simulink model "force_control"  (R2021a)
settings: Solver=FixedStepDiscrete  StartTime=0.0  StopTime=inf  FixedStep=0.001  RelTol=1e-3  EnableMultiTasking=on
PreLoadFcn:
  | demos_common_configs();
undefined symbols (not defined in the file): ddQ2_desired, ddQ4_desired, DiscIntNeverNeededParam, dQ2_desired, dQ4_desired, Q2_desired, Q4_desired, T
libraries: simulink x6, franka_simulink_library_misc x5, franka_simulink_library x4
settings Model: SimulationMode=external  ExtModeTrigDuration=10000  Creator=vasi_ko  LastModifiedBy=robohub
settings SolverCC: AlgebraicLoopSolver=TrustRegion
settings DataIOCC: LimitDataPoints=on  SaveFormat=Array  ReturnWorkspaceOutputs=off
settings OptimizationCC: DefaultParameterBehavior=Inlined  EnhancedBackFolding=on  PassReuseOutputArgsAs=Individual arguments  ZeroExternalMemoryAtStartup=off  ZeroInternalMemoryAtStartup=off  OptimizeBlockOrder=speed  DifferentSizesBufferReuse=on  OptimizationCustomize=off  EfficientTunableParamExpr=on
settings DebuggingCC: SolverPrmCheckMsg=warning  ParameterTunabilityLossMsg=error  SFUnexpectedBacktrackingDiag=warning  SFNoUnconditionalDefaultTransitionDiag=warning  SFExecutionAtInitializationDiag=none  SFMachineParentedDataDiag=warning  ArithmeticOperatorsInVariantConditions=warning
settings HardwareCC: ProdBitPerLong=64  ProdHWDeviceType=Intel->x86-64 (Linux 64)
settings ModelReferenceCC: PropagateSignalLabelsOutOfModel=off
settings SFSimCC: SimUseLocalCustomCode=off  MATLABDynamicMemAlloc=off  CustomCodeUndefinedFunction=UseInterfaceOnly  SimTargetLang=C++
settings RTWCC: SystemTargetFile=franka_emika_panda.tlc  GenCodeOnly=on  TemplateMakefile=ert_default_tmf  RTWVerbose=off  RTWUseLocalCustomCode=off  Toolchain=Franka Simulink | gmake (64-bit linux)  BuildConfiguration=Faster Runs  IncludeHyperlinkInReport=on  TargetLang=C++
settings CodeAppCC: ForceParamTrailComments=on  IgnoreCustomStorageClasses=off  OperatorAnnotations=on  SimulinkDataObjDesc=on  SFDataObjDesc=on  InsertBlockDesc=on
settings STFCustomTargetCC: TargetLangStandard=C99 (ISO)  MultiwordLength=256  GenerateSampleERTMain=on  ModelReferenceCompliant=off  CombineOutputUpdateFcns=on  ERTCustomFileBanners=on  SupportNonInlinedSFcns=off  RemoveResetFunc=on  MATLABClassNameForMDSCustomization=Simulink.SoftwareTarget.ERTCustomization  CPPClassGenCompliant=on  GRTInterface=off  SystemTargetFile=franka_emika_panda.tlc
settings ERTTargetCC: TargetLangStandard=C99 (ISO)  GenerateSampleERTMain=on  ModelReferenceCompliant=off  ParMdlRefBuildCompliant=off  CompOptLevelCompliant=off  ConcurrentExecutionCompliant=off  SupportContinuousTime=on  ModelStepFunctionPrototypeControlCompliant=off  ExtMode=on  ExtModeMexArgs='129.97.71.27' 0 17725  InlinedParameterPlacement=NonHierarchical  ERTCustomFileTemplate=franka_emika_panda_file_process.tlc
settings ConfigComp: CovMetricSettings=dw  CovSaveCumulativeToWorkspaceVar=on  CovSaveSingleToWorkspaceVar=on  CovExternalEMLEnable=off  CovSFcnEnable=off

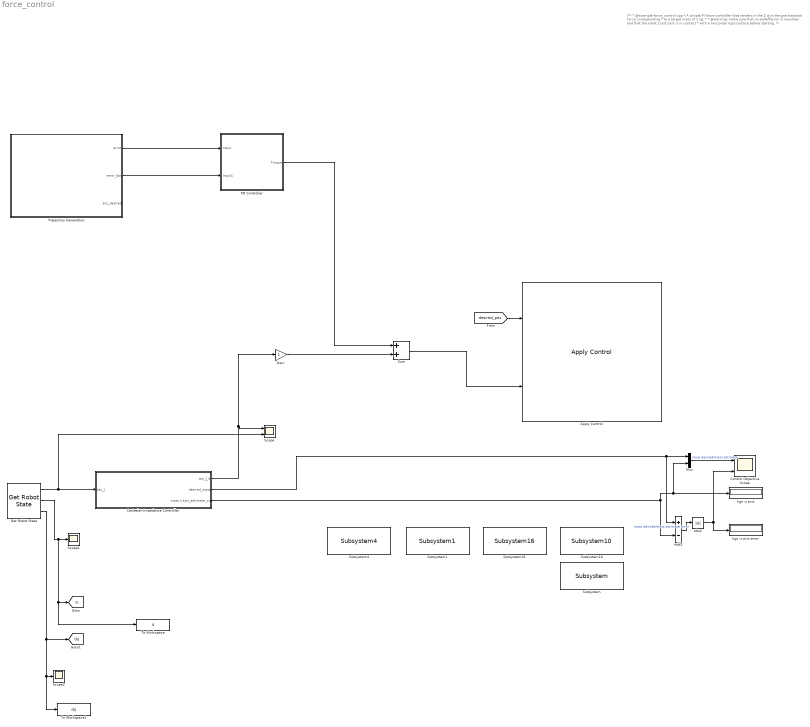
== system force_control ==
  note: /**
      |  * @example force_control.cpp
      |  * A simple PI force controller that renders in the Z axis the gravitational force corresponding
      |  * to a target mass of 1 kg.
      |  *
      |  * @warning: make sure that no endeffector is mounted and that the robot's last joint is in contact
      |  * with a horizontal rigid surface before starting.
      |  */
  Abs2 : Abs
  Add1 : Sum  Inputs=+-
  Apply Control : franka_simulink_library/Apply Control  robot_ip=robot_ip  gripper_attached=off  control_mode=Torque Control - Joint Positions  controller_choice=Joint Impedance Controller  elbow_control=on  collision_thresholds=100*ones(1,52)  joint_impedance=joint_impedance  cartesian_impedance=cartesian_impedance  load_inertia=load_inertia  EE_T_K=EE_T_K  init_joint_configuration_req=off  init_joint_configuration=[0.00392584915725334;-0.104076810189763;0.0404703493577216;-2.7334242600631;0.0113035300040543;2.63364770337236;0.372162046953987]
      settings: SourceProductName=Franka Emika
  Cartesian Impedance Controller : Subsystem
      mask Display:
      | disp('{\bf\fontsize{18}Force Controller}', 'texmode','on');
      | %
      | % block_icon('Controller')
      | %
      | port_label('input',1,'tau_J');
      | port_label('output',1,'tau_J_d');
      | port_label('output',2,'mass desired');
      | port_label('output',3,'mass estimate');
  Control Objective Scope : Scope  NumInputPorts=2
  Gain : Gain
  Get Robot State : franka_simulink_library/Get Robot State  robot_ip=robot_ip  signals_requested='tau_J q dq'
      settings: SourceProductName=Franka Emika
  Mux : Mux  Inputs=2
  PD Controller : Subsystem
  Scope : Scope  NumInputPorts=2
  Scope1 : Scope
  Scope2 : Scope
  Subsystem : franka_simulink_library_misc/Subsystem  SystemSampleTime=-1  VariantActivationTime=update diagram  Latency=0  AutoFrameSizeCalculation=off
  Subsystem1 : franka_simulink_library_misc/Subsystem1  SystemSampleTime=-1  VariantActivationTime=update diagram  Latency=0  AutoFrameSizeCalculation=off
  Subsystem10 : franka_simulink_library_misc/Subsystem10  SystemSampleTime=-1  VariantActivationTime=update diagram  Latency=0  AutoFrameSizeCalculation=off
  Subsystem16 : franka_simulink_library_misc/Subsystem16  SystemSampleTime=-1  VariantActivationTime=update diagram  Latency=0  AutoFrameSizeCalculation=off
  Subsystem4 : franka_simulink_library_misc/Subsystem4  SystemSampleTime=-1  VariantActivationTime=update diagram  Latency=0  AutoFrameSizeCalculation=off
  Sum : Sum
  To Workspace : ToWorkspace  VariableName=q  SaveFormat=Structure With Time  SampleTime=-1
  To Workspace1 : ToWorkspace  VariableName=dq  SaveFormat=Structure With Time  SampleTime=-1
  Trajectory Generation : Subsystem
  kgs -z axis : Display
  kgs -z axis error : Display
  tag scope: dq=global, q=global
  wires:
  Get Robot State/1 -> Scope/2, Cartesian Impedance Controller/1(tau_J)
  Mux/1 -> Control Objective Scope/1  "mass desired/mass estimate"
  Cartesian Impedance Controller/1(tau_J_d) -> Gain/1, Scope/1
  Cartesian Impedance Controller/2(desired_mass) -> Add1/1, Mux/1
  Cartesian Impedance Controller/3(mass z axis_estimate_out) -> kgs -z axis/1, Mux/2, Add1/2
  Add1/1 -> Abs2/1  "mass desired/mass estimate error"
  Abs2/1 -> kgs -z axis error/1, Control Objective Scope/2
  Get Robot State/3 -> [dq], To Workspace1/1, Scope2/1
  Trajectory Generation/2(error_dot) -> PD Controller/2(Input1)
  Trajectory Generation/1(error) -> PD Controller/1(Input)
  Get Robot State/2 -> [q], To Workspace/1, Scope1/1
  PD Controller/1(Torque) -> Sum/1
  Gain/1 -> Sum/2
  Sum/1 -> Apply Control/2
  [desired_pos] -> Apply Control/1

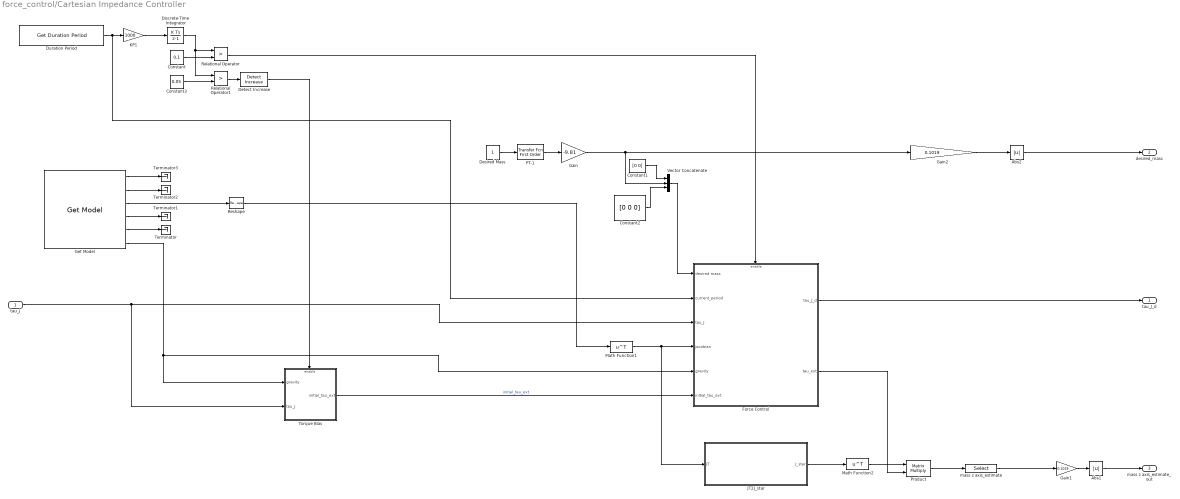
== system force_control/Cartesian Impedance Controller ==
  tau_J : Inport
  Abs1 : Abs
  Abs2 : Abs
  Constant : Constant  Value=0.1
  Constant1 : Constant  Value=[0 0]
  Constant2 : Constant  Value=[0 0 0]
  Constant3 : Constant  Value=0.05
  Desired Mass : Constant
  Detect Increase : simulink/Logic and Bit Operations/Detect Increase  vinit=0.0  OutDataTypeStr=boolean
  Discrete-Time Integrator : DiscreteIntegrator  SampleTime=-1  ICPrevOutput=DiscIntNeverNeededParam  ICPrevScaledInput=DiscIntNeverNeededParam
  Duration Period : franka_simulink_library/Get Duration Period  robot_ip=robot_ip
      settings: SourceProductName=Franka Emika
  Force Control : Subsystem
  Gain : Gain  Gain=-9.81
  Gain1 : Gain  Gain=0.1019
  Gain2 : Gain  Gain=0.1019
  Get Model : franka_simulink_library/Get Model  robot_ip=robot_ip
      settings: SourceProductName=Franka Emika
  JT2J_star : MATLAB Function  TreatAsAtomicUnit=on
  KP1 : Gain  Gain=1000
  Math Function1 : Math  Operator=transpose  SignedPower=on  SaturateOnIntegerOverflow=on
  Math Function2 : Math  Operator=transpose  SignedPower=on  SaturateOnIntegerOverflow=on
  PT-1 : simulink/Discrete/Transfer Fcn First Order  PoleZ=0.9988  ICPrevOutput=0.0  DoSatur=off
  Product : Product  Multiplication=Matrix(*)
  Relational Operator : RelationalOperator  Operator=>  OutDataTypeStr=boolean  RndMeth=Nearest
  Relational Operator1 : RelationalOperator  Operator=>  OutDataTypeStr=boolean  RndMeth=Nearest
  Reshape : Reshape  OutputDimensionality=Customize  OutputDimensions=[6,7]
  Terminator{,1..3} (4 alike) : Terminator
  Torque Bias : Subsystem
  Vector Concatenate : Concatenate  NumInputs=3
  mass z axis_estimate : Selector  InputPortWidth=6  IndexOptions=Index vector (dialog)  Indices=3  OutputSizes=1
  tau_J_d : Outport  VectorParamsAs1DForOutWhenUnconnected=off
  desired_mass : Outport  Port=2  VectorParamsAs1DForOutWhenUnconnected=off
  mass z axis_estimate_out : Outport  Port=3  VectorParamsAs1DForOutWhenUnconnected=off
  wires:
  Get Model/5 -> Terminator/1
  Get Model/4 -> Terminator1/1
  Get Model/3 -> Reshape/1
  tau_J/1 -> Force Control/3(tau_J), Torque Bias/2(tau_J)
  Discrete-Time Integrator/1 -> Relational Operator1/1, Relational Operator/1
  Constant/1 -> Relational Operator/2
  KP1/1 -> Discrete-Time Integrator/1
  Constant1/1 -> Vector Concatenate/1
  Constant2/1 -> Vector Concatenate/3
  Desired Mass/1 -> PT-1/1
  Gain/1 -> Vector Concatenate/2, Gain2/1
  Force Control/1(tau_J_d) -> tau_J_d/1
  Torque Bias/1(initial_tau_ext) -> Force Control/6(initial_tau_ext)  "initial_tau_ext"
  Get Model/6 -> Torque Bias/1(gravity), Force Control/5(gravity)
  Relational Operator/1 -> Force Control/Enable
  Reshape/1 -> Math Function1/1
  Duration Period/1 -> KP1/1, Force Control/2(current_period)
  Constant3/1 -> Relational Operator1/2
  Relational Operator1/1 -> Detect Increase/1
  Detect Increase/1 -> Torque Bias/Enable
  Vector Concatenate/1 -> Force Control/1(desired mass)
  PT-1/1 -> Gain/1
  Force Control/2(tau_ext) -> Product/2
  Gain1/1 -> Abs1/1
  Gain2/1 -> Abs2/1
  Abs1/1 -> mass z axis_estimate_out/1
  Abs2/1 -> desired_mass/1
  Get Model/1 -> Terminator3/1
  mass z axis_estimate/1 -> Gain1/1
  Get Model/2 -> Terminator2/1
  Product/1 -> mass z axis_estimate/1
  Math Function1/1 -> JT2J_star/1(JT), Force Control/4(Jacobian)
  JT2J_star/1(J_star) -> Math Function2/1
  Math Function2/1 -> Product/1

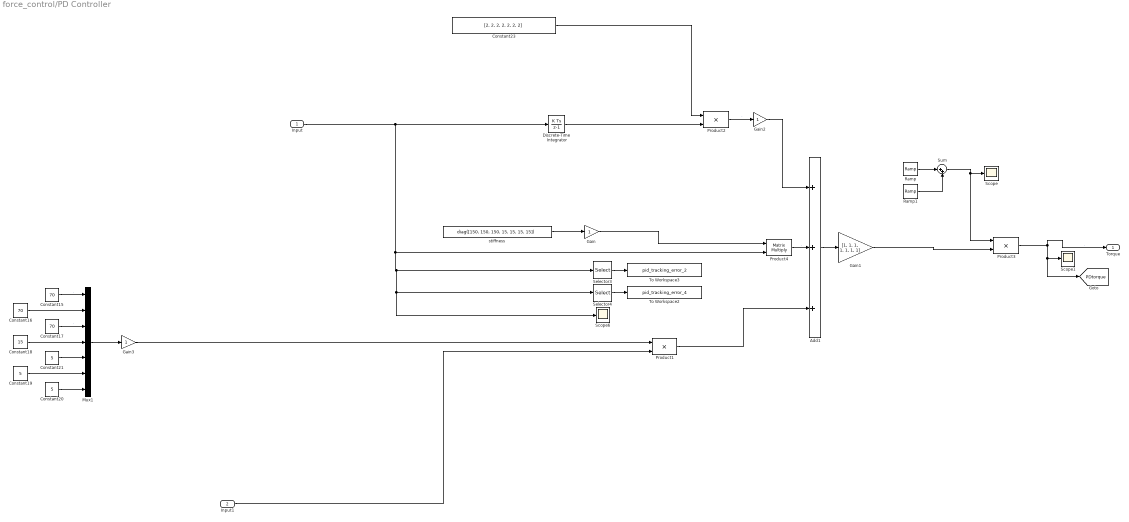
== system force_control/PD Controller ==
  Input : Inport
  Input1 : Inport  Port=2
  Add1 : Sum  Inputs=+++
  Constant15 : Constant  Value=70
  Constant16 : Constant  Value=70
  Constant17 : Constant  Value=70
  Constant18 : Constant  Value=15
  Constant19 : Constant  Value=5
  Constant20 : Constant  Value=5
  Constant21 : Constant  Value=5
  Constant23 : Constant  Value=[2, 2, 2, 2, 2, 2, 2]
  Discrete-Time Integrator : DiscreteIntegrator  SampleTime=-1  ICPrevOutput=DiscIntNeverNeededParam  ICPrevScaledInput=DiscIntNeverNeededParam
  Gain : Gain
  Gain1 : Gain  Gain=[1, 1, 1, 1, 1, 1, 1]
  Gain2 : Gain
  Gain3 : Gain
  Mux1 : Mux  Inputs=7
  Product1 : Product
  Product2 : Product
  Product3 : Product
  Product4 : Product  Multiplication=Matrix(*)
  Ramp : simulink/Sources/Ramp  slope=0.1  start=0  InitialOutput=0
  Ramp1 : simulink/Sources/Ramp  slope=-0.1  start=10  InitialOutput=0
  Scope : Scope
  Scope1 : Scope
  Scope6 : Scope
  Selector3 : Selector  InputPortWidth=7  IndexOptions=Index vector (dialog)  Indices=[2]  OutputSizes=1
  Selector4 : Selector  InputPortWidth=7  IndexOptions=Index vector (dialog)  Indices=[4]  OutputSizes=1
  Sum : Sum  Inputs=|++
  To Workspace2 : ToWorkspace  VariableName=pid_tracking_error_4  SaveFormat=Structure With Time  SampleTime=-1
  To Workspace3 : ToWorkspace  VariableName=pid_tracking_error_2  SaveFormat=Structure With Time  SampleTime=-1
  stiffness : Constant  Value=diag([150, 150, 150, 15, 15, 15, 15])  VectorParams1D=off
  Torque : Outport
  tag scope: PDtorque=global
  wires:
  Product4/1 -> Add1/2  "."
  Mux1/1 -> Gain3/1
  Constant16/1 -> Mux1/2
  Constant18/1 -> Mux1/4
  Constant19/1 -> Mux1/6
  Constant20/1 -> Mux1/7
  Constant21/1 -> Mux1/5
  Constant15/1 -> Mux1/1  "."
  Constant17/1 -> Mux1/3  "."
  Product1/1 -> Add1/3
  Add1/1 -> Gain1/1
  Constant23/1 -> Product2/1
  Product2/1 -> Gain2/1  "."
  Discrete-Time Integrator/1 -> Product2/2
  Selector4/1 -> To Workspace2/1
  Selector3/1 -> To Workspace3/1
  stiffness/1 -> Gain/1
  Gain2/1 -> Add1/1
  Gain3/1 -> Product1/1
  Input/1 -> Scope6/1, Selector4/1, Selector3/1, Product4/2, Discrete-Time Integrator/1
  Input1/1 -> Product1/2
  Gain/1 -> Product4/1
  Ramp/1 -> Sum/1
  Ramp1/1 -> Sum/2
  Gain1/1 -> Product3/2
  Product3/1 -> Torque/1, Scope1/1, [PDtorque]  "."
  Sum/1 -> Scope/1, Product3/1

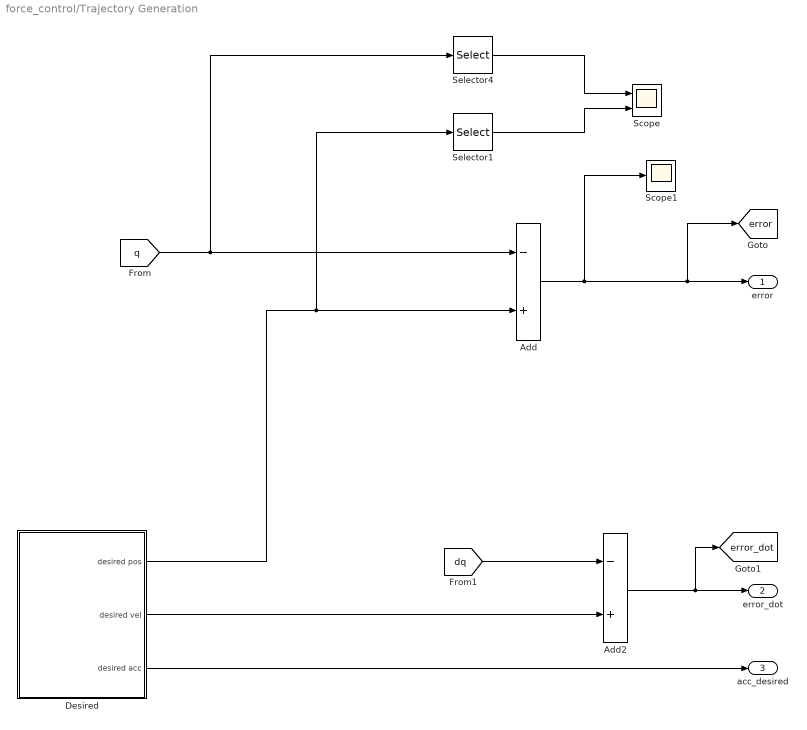
== system force_control/Trajectory Generation ==
  Add : Sum  Inputs=-+
  Add2 : Sum  Inputs=-+
  Desired : Subsystem
  Scope : Scope  NumInputPorts=2
  Scope1 : Scope
  Selector1 : Selector  InputPortWidth=7  IndexOptions=Index vector (dialog)  Indices=[6]  OutputSizes=1
  Selector4 : Selector  InputPortWidth=7  IndexOptions=Index vector (dialog)  Indices=[6]  OutputSizes=1
  error : Outport
  error_dot : Outport  Port=2
  acc_desired : Outport  Port=3
  tag scope: error=global, error_dot=global
  wires:
  Desired/2(desired vel) -> Add2/2
  Desired/1(desired pos) -> Selector1/1, Add/2
  Add/1 -> Scope1/1, error/1, [error]
  Add2/1 -> [error_dot], error_dot/1
  Desired/3(desired acc) -> acc_desired/1
  [dq] -> Add2/1
  Selector4/1 -> Scope/1
  Selector1/1 -> Scope/2
  [q] -> Selector4/1, Add/1

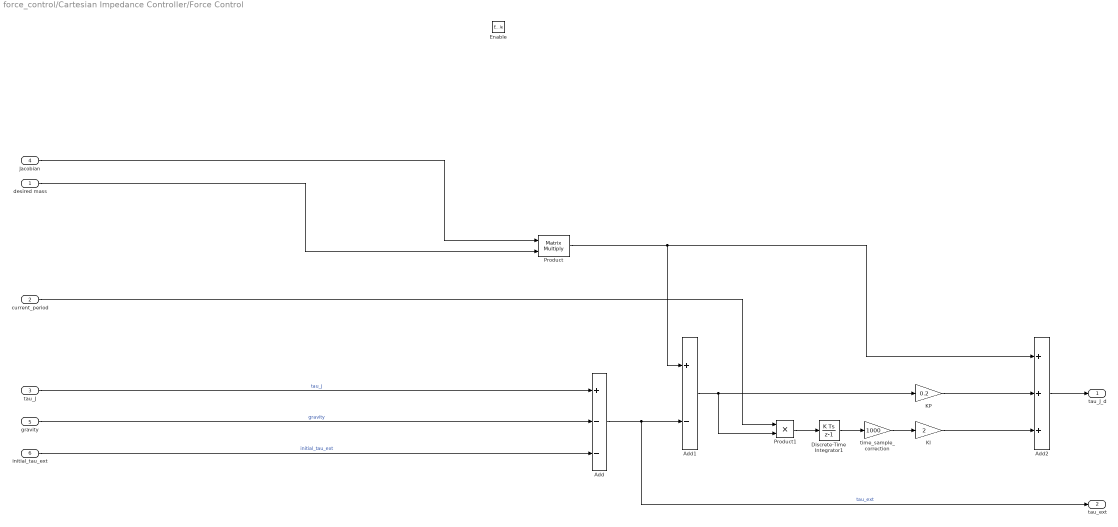
== system force_control/Cartesian Impedance Controller/Force Control ==
  desired mass : Inport
  current_period : Inport  Port=2
  tau_J : Inport  Port=3
  Jacobian : Inport  Port=4
  gravity : Inport  Port=5
  initial_tau_ext : Inport  Port=6
  Enable : EnablePort
  Add : Sum  Inputs=+--
  Add1 : Sum  Inputs=+-
  Add2 : Sum  Inputs=+++
  Discrete-Time Integrator1 : DiscreteIntegrator  SampleTime=0.001  ICPrevOutput=DiscIntNeverNeededParam  ICPrevScaledInput=DiscIntNeverNeededParam
  KI : Gain  Gain=2
  KP : Gain  Gain=0.2
  Product : Product  Multiplication=Matrix(*)
  Product1 : Product
  time_sample_correction : Gain  Gain=1000
  tau_J_d : Outport  InitialOutput=[0 0 0 0 0 0 0]  VectorParamsAs1DForOutWhenUnconnected=off
  tau_ext : Outport  Port=2  InitialOutput=[0 0 0 0 0 0 0]  VectorParamsAs1DForOutWhenUnconnected=off
  wires:
  Jacobian/1 -> Product/1
  tau_J/1 -> Add/1  "tau_J"
  gravity/1 -> Add/2  "gravity"
  Add/1 -> tau_ext/1, Add1/2  "tau_ext"
  Add1/1 -> Product1/2, KP/1
  Add2/1 -> tau_J_d/1
  Product1/1 -> Discrete-Time Integrator1/1
  current_period/1 -> Product1/1
  KI/1 -> Add2/3
  initial_tau_ext/1 -> Add/3  "initial_tau_ext"
  Product/1 -> Add1/1, Add2/1
  KP/1 -> Add2/2
  desired mass/1 -> Product/2
  Discrete-Time Integrator1/1 -> time_sample_correction/1
  time_sample_correction/1 -> KI/1

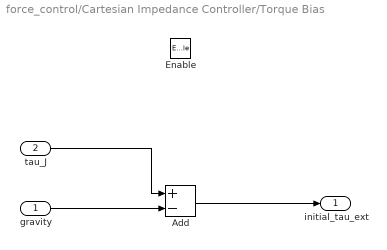
== system force_control/Cartesian Impedance Controller/Torque Bias ==
  gravity : Inport
  tau_J : Inport  Port=2
  Enable : EnablePort
  Add : Sum  Inputs=+-
  initial_tau_ext : Outport  InitialOutput=[0 0 0 0 0 0 0]  VectorParamsAs1DForOutWhenUnconnected=off
  wires:
  tau_J/1 -> Add/1
  gravity/1 -> Add/2
  Add/1 -> initial_tau_ext/1

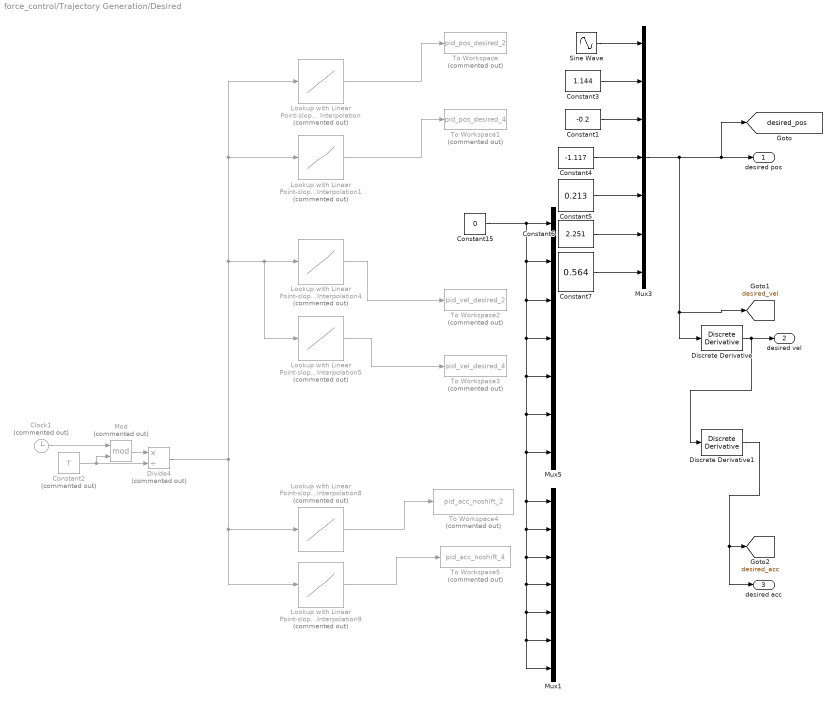
== system force_control/Trajectory Generation/Desired ==
  Clock1 : Clock  Commented=on
  Constant1 : Constant  Value=-0.2
  Constant15 : Constant  Value=0
  Constant2 : Constant  Commented=on  Value=T
  Constant3 : Constant  Value=1.144
  Constant4 : Constant  Value=-1.117
  Constant5 : Constant  Value=0.213
  Constant6 : Constant  Value=2.251
  Constant7 : Constant  Value=0.564
  Discrete Derivative : simulink/Discrete/Discrete Derivative  gainval=1.0  ICPrevScaledInput=0.0  OutMin=[]  OutMax=[]  OutDataType=fixdt(1, 16)  OutScaling=2^-10  DoSatur=off
  Discrete Derivative1 : simulink/Discrete/Discrete Derivative  gainval=1.0  ICPrevScaledInput=0.0  OutMin=[]  OutMax=[]  OutDataType=fixdt(1, 16)  OutScaling=2^-10  DoSatur=off
  Divide4 : Product  Commented=on  Inputs=*/
  Lookup with Linear Point-slope Interpolation : Lookup_n-D  Commented=on  NumberOfTableDimensions=1  BreakpointsForDimension1=linspace(0,1,length(Q2_desired))  Table=Q2_desired  InternalRulePriority=Speed  RndMeth=Simplest  InputSameDT=on
  Lookup with Linear Point-slope Interpolation1 : Lookup_n-D  Commented=on  NumberOfTableDimensions=1  BreakpointsForDimension1=linspace(0,1,length(Q4_desired))  Table=Q4_desired  InternalRulePriority=Speed  RndMeth=Simplest  InputSameDT=on
  Lookup with Linear Point-slope Interpolation4 : Lookup_n-D  Commented=on  NumberOfTableDimensions=1  BreakpointsForDimension1=linspace(0,1,length(dQ2_desired))  Table=dQ2_desired  InternalRulePriority=Speed  RndMeth=Simplest  InputSameDT=on
  Lookup with Linear Point-slope Interpolation5 : Lookup_n-D  Commented=on  NumberOfTableDimensions=1  BreakpointsForDimension1=linspace(0,1,length(dQ4_desired))  Table=dQ4_desired  InternalRulePriority=Speed  RndMeth=Simplest  InputSameDT=on
  Lookup with Linear Point-slope Interpolation8 : Lookup_n-D  Commented=on  NumberOfTableDimensions=1  BreakpointsForDimension1=linspace(0,1,length(ddQ2_desired))  Table=ddQ2_desired  InternalRulePriority=Speed  RndMeth=Simplest  InputSameDT=on
  Lookup with Linear Point-slope Interpolation9 : Lookup_n-D  Commented=on  NumberOfTableDimensions=1  BreakpointsForDimension1=linspace(0,1,length(ddQ2_desired))  Table=ddQ4_desired  InternalRulePriority=Speed  RndMeth=Simplest  InputSameDT=on
  Mod : Math  Commented=on  Operator=mod  SaturateOnIntegerOverflow=on
  Mux1 : Mux  Inputs=7
  Mux3 : Mux  Inputs=7
  Mux5 : Mux  Inputs=7
  Sine Wave : Sin  Amplitude=0.6  Bias=0.6  SampleTime=0
  To Workspace : ToWorkspace  Commented=on  VariableName=pid_pos_desired_2  SaveFormat=Structure With Time  SampleTime=-1
  To Workspace1 : ToWorkspace  Commented=on  VariableName=pid_pos_desired_4  SaveFormat=Structure With Time  SampleTime=-1
  To Workspace2 : ToWorkspace  Commented=on  VariableName=pid_vel_desired_2  SaveFormat=Structure With Time  SampleTime=-1
  To Workspace3 : ToWorkspace  Commented=on  VariableName=pid_vel_desired_4  SaveFormat=Structure With Time  SampleTime=-1
  To Workspace4 : ToWorkspace  Commented=on  VariableName=pid_acc_noshift_2  SaveFormat=Structure With Time  SampleTime=-1
  To Workspace5 : ToWorkspace  Commented=on  VariableName=pid_acc_noshift_4  SaveFormat=Structure With Time  SampleTime=-1
  desired pos : Outport
  desired vel : Outport  Port=2
  desired acc : Outport  Port=3
  tag scope: desired_acc=global, desired_pos=global, desired_vel=global
  wires:
  Lookup with Linear Point-slope Interpolation4/1 -> To Workspace2/1
  Constant15/1 -> Mux5/2, Mux5/3, Mux5/4, Mux5/5, Mux5/6, Mux5/7, Mux1/2, Mux1/7, Mux1/6, Mux1/5, Mux1/4, Mux1/3, Mux1/1, Mux5/1
  Clock1/1 -> Mod/1
  Lookup with Linear Point-slope Interpolation1/1 -> To Workspace1/1
  Lookup with Linear Point-slope Interpolation8/1 -> To Workspace4/1
  Lookup with Linear Point-slope Interpolation/1 -> To Workspace/1
  Lookup with Linear Point-slope Interpolation5/1 -> To Workspace3/1
  Constant6/1 -> Mux3/6
  Constant5/1 -> Mux3/5
  Constant1/1 -> Mux3/3
  Divide4/1 -> Lookup with Linear Point-slope Interpolation/1, Lookup with Linear Point-slope Interpolation1/1, Lookup with Linear Point-slope Interpolation5/1, Lookup with Linear Point-slope Interpolation4/1, Lookup with Linear Point-slope Interpolation9/1, Lookup with Linear Point-slope Interpolation8/1
  Constant7/1 -> Mux3/7
  Lookup with Linear Point-slope Interpolation9/1 -> To Workspace5/1
  Sine Wave/1 -> Mux3/1
  Mux3/1 -> [desired_vel], Discrete Derivative/1, [desired_pos], desired pos/1
  Constant2/1 -> Mod/2, Divide4/2
  Mod/1 -> Divide4/1
  Constant3/1 -> Mux3/2
  Constant4/1 -> Mux3/4
  Discrete Derivative/1 -> Discrete Derivative1/1, desired vel/1
  Discrete Derivative1/1 -> [desired_acc], desired acc/1

== matlab function force_control/Cartesian Impedance Controller/JT2J_star ==
  data: JT input; J_star output
function J_star = JT2J_star(JT)
%#codegen

J = JT';
% low isotropic damping, the value should be much smaller than lambda_max^2
beta =0;
% damping added in singular directions, we chose it to be equal to
% threshold
% lambda_max = singularity_threshold_inverse_kinematics; 
% SVD decomposition
[U,S,~] = svd(J);
sigma = diag(S);
% rank
singularity_threshold_inverse_kinematics = eps;
r = sum(sigma > singularity_threshold_inverse_kinematics);
% initilizing damping
  lambda_square_vector = zeros(6,1);
if r==6 % damping in full rank case is zero
    lambda_square_vector = zeros(6,1);
else % daamping in rank deficient cases
%     sigma_singular = sigma(r+1:6);
%     lambda_square_vector(r+1:6) = ...
%         (1 - (sigma_singular/ singularity_threshold_inverse_kinematics).^2) *...
%         lambda_max^2;
end
J_star =  JT * U * diag(1./(sigma.^2+lambda_square_vector+beta^2*ones(6,1)))*U';

end
